simulink model "kfs_pr_1"  (R2019a)
settings: Solver=FixedStepAuto  StartTime=0.0  StopTime=10000  FixedStep=1  RelTol=1e-3
values from neighbouring files (symbols this model uses):
  mb = 10800    [params.m]
  min_paus = 100    [params.m]
  nurk = deg2rad(0)    [params.m]
  vy_0 = 0    [params.m]
  x_0 = 0    [params.m]
  y_0 = 0    [params.m]
libraries: dspswit3 x1, simulink x1
settings Model: Creator=Kasutaja  LastModifiedBy=Kasutaja
settings DataIOCC: ReturnWorkspaceOutputs=off
settings DebuggingCC: ArithmeticOperatorsInVariantConditions=warning

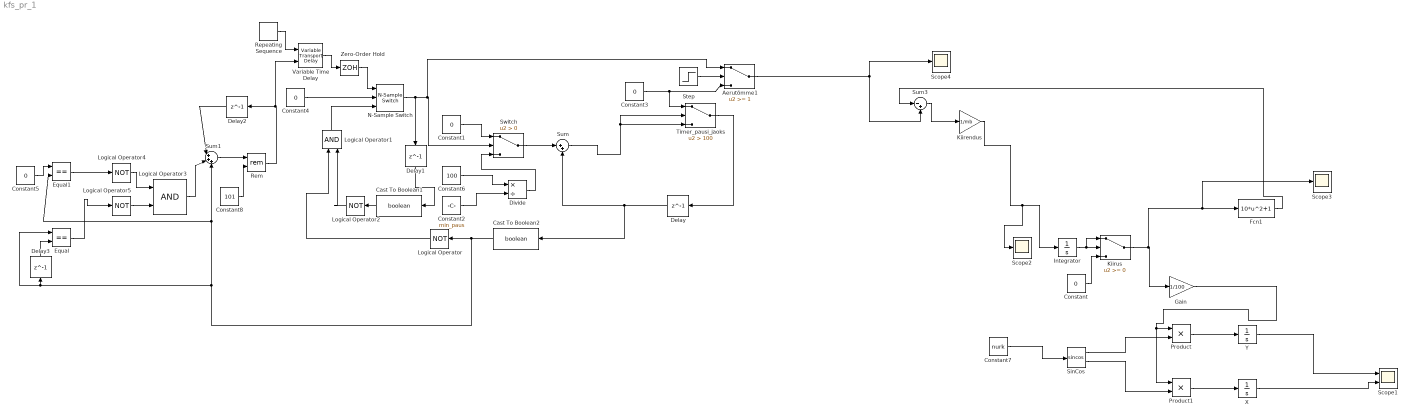
== system kfs_pr_1 ==
  Aerutõmme1 : Switch  Threshold=1
  Cast To Boolean1 : DataTypeConversion  OutDataTypeStr=boolean
  Cast To Boolean2 : DataTypeConversion  OutDataTypeStr=boolean
  Constant{,1,3..5} (5 alike) : Constant  Value=0
  Constant2 : Constant  Value=min_paus  SampleTime=1
  Constant6 : Constant  Value=100  SampleTime=1
  Constant7 : Constant  Value=nurk
  Constant8 : Constant  Value=101
  Delay{,1..3} (4 alike) : Delay  DelayLength=1  InitialCondition=0
  Divide : Product  Inputs=*/
  Equal : RelationalOperator  Operator===  OutDataTypeStr=boolean  RndMeth=Simplest
  Equal1 : RelationalOperator  Operator===  OutDataTypeStr=boolean  RndMeth=Simplest
  Fcn1 : Fcn  Expr=10*u^2+1
  Gain : Gain  Gain=1/100
  Integrator : Integrator  InitialCondition=vy_0
  Kiirendus : Gain  Gain=1/mb
  Kiirus : Switch
  Logical Operator{,2,4..5} (4 alike) : Logic  Operator=NOT  IconShape=distinctive  AllPortsSameDT=off  OutDataTypeStr=boolean
  Logical Operator1 : Logic  IconShape=distinctive  AllPortsSameDT=off  OutDataTypeStr=boolean
  Logical Operator3 : Logic  IconShape=distinctive  AllPortsSameDT=off  OutDataTypeStr=boolean
  N-Sample Switch : dspswit3/N-Sample Switch  N=101  reset=on  TriggerType=Non-zero sample  Ts=1
      settings: SourceProductName=DSP System Toolbox  SourceProductBaseCode=DS
  Product : Product
  Product1 : Product
  Rem : Math  Operator=rem  SaturateOnIntegerOverflow=on
  Repeating Sequence : simulink/Sources/Repeating Sequence  rep_seq_t=|  rep_seq_y=|
      rep_seq_t=|
      | [0
      | 1
      | 2
      | 3
      | 4
      | 5
      | 6
      | 7
      | 8
      | 9
      | 10
      | 11
      | 12
      | 13
      | 14
      | 15
      | 16
      | 17
      | 18
      | 19
      | 20
      | 21
      | 22
      | 23
      | 24
      | 25
      | 26
      | 27
      | 28
      | 29
      | 30
      | 31
      | 32
      | 33
      | 34
      | 35
      | 36
      | 37
      | 38
      | 39
      | 40
      | 41
      | 42
      | 43
      | 44
      | 45
      | 46
      | 47
      | 48
      | 49
      | 50
      | 51
      | 52
      | 53
      | 54
      | 55
      | 56
      | 57
      | 58
      | 59
      | 60
      | 61
      | 62
      | 63
      | 64
      | 65
      | 66
      | 67
      | 68
      | 69
      | 70
      | 71
      | 72
      | 73
      | 74
      | 75
      | 76
      | 77
      | 78
      | 79
      | 80
      | 81
      | 82
      | 83
      | 84
      | 85
      | 86
      | 87
      | 88
      | 89
      | 90
      | 91
      | 92
      | 93
      | 94
      | 95
      | 96
      | 97
      | 98
      | 99
      | 100
      | 101  ]
      rep_seq_y=|
      | [1
      | 14
      | 28
      | 42
      | 56
      | 70
      | 84
      | 98
      | 112
      | 126
      | 167
      | 208
      | 249
      | 290
      | 331
      | 372
      | 413
      | 454
      | 495
      | 536
      | 551
      | 566
      | 581
      | 596
      | 611
      | 626
      | 641
      | 656
      | 671
      | 686
      | 697
      | 708
      | 719
      | 730
      | 741
      | 752
      | 763
      | 774
      | 785
      | 796
      | 801
      | 806
      | 811
      | 816
      | 821
      | 826
      | 831
      | 836
      | 841
      | 846
      | 841
      | 836
      | 831
      | 826
      | 821
      | 816
      | 811
      | 806
      | 801
      | 796
      | 785
      | 774
      | 763
      | 752
      | 741
      | 730
      | 719
      | 708
      | 697
      | 686
      | 646
      | 606
      | 566
      | 526
      | 486
      | 446
      | 406
      | 366
      | 326
      | 286
      | 279
      | 272
      | 265
      | 258
      | 251
      | 244
      | 237
      | 230
      | 223
      | 216
      | 198
      | 180
      | 162
      | 144
      | 126
      | 108
      | 90
      | 72
      | 54
      | 36
      | 18
      | -1  ]
  Scope1 : Scope  NumInputPorts=2
  Scope2 : Scope
  Scope3 : Scope
  Scope4 : Scope
  SinCos : Trigonometry  Operator=sincos
  Step : Step  Time=2000  Before=1  After=0  SampleTime=1
  Sum : Sum  Inputs=|++
  Sum1 : Sum  Inputs=|+++
  Sum3 : Sum  Inputs=|-+
  Switch : Switch  Criteria=u2 > Threshold
  Timer_pausi_jaoks : Switch  Criteria=u2 > Threshold  Threshold=100
  Variable Time Delay : VariableTransportDelay  MaximumDelay=200  MaximumPoints=256  ZeroDelay=on
  X : Integrator  InitialCondition=x_0
  Y : Integrator  InitialCondition=y_0
  Zero-Order Hold : ZeroOrderHold
  wires:
  Aerutõmme1/1 -> Sum3/2, Scope4/1
  X/1 -> Scope1/2
  Fcn1/1 -> Sum3/1
  Y/1 -> Scope1/1
  Product1/1 -> X/1
  Constant7/1 -> SinCos/1
  Kiirendus/1 -> Integrator/1, Scope2/1
  SinCos/1 -> Product/2
  SinCos/2 -> Product1/2
  Product/1 -> Y/1
  Gain/1 -> Product1/1, Product/1
  Sum3/1 -> Kiirendus/1
  Cast To Boolean2/1 -> Sum1/3, Equal1/2, Delay3/1, Equal/1, Logical Operator/1
  Constant6/1 -> Divide/1
  Constant5/1 -> Equal1/1
  Logical Operator1/1 -> N-Sample Switch/3
  Constant1/1 -> Switch/1
  Zero-Order Hold/1 -> N-Sample Switch/1
  Repeating Sequence/1 -> Variable Time Delay/1
  Logical Operator5/1 -> Logical Operator3/2
  Constant3/1 -> Aerutõmme1/3, Timer_pausi_jaoks/1
  Delay1/1 -> Cast To Boolean1/1
  Constant2/1 -> Divide/2
  Logical Operator3/1 -> Sum1/2
  Delay/1 -> Cast To Boolean2/1, Sum/2
  Equal/1 -> Logical Operator5/1
  Step/1 -> Aerutõmme1/2
  Timer_pausi_jaoks/1 -> Delay/1
  Delay3/1 -> Equal/2
  Sum/1 -> Timer_pausi_jaoks/3, Timer_pausi_jaoks/2
  Sum1/1 -> Rem/1
  Divide/1 -> Switch/3
  Delay2/1 -> Sum1/1
  Equal1/1 -> Logical Operator4/1
  Logical Operator/1 -> Logical Operator1/1
  Constant4/1 -> N-Sample Switch/2
  Switch/1 -> Sum/1
  Logical Operator4/1 -> Logical Operator3/1
  Logical Operator2/1 -> Logical Operator1/2
  Cast To Boolean1/1 -> Logical Operator2/1
  Kiirus/1 -> Scope3/1, Fcn1/1, Gain/1
  Integrator/1 -> Kiirus/1, Kiirus/2
  Constant/1 -> Kiirus/3
  Rem/1 -> Variable Time Delay/2, Delay2/1
  Constant8/1 -> Rem/2
  Variable Time Delay/1 -> Zero-Order Hold/1
  N-Sample Switch/1 -> Aerutõmme1/1, Switch/2, Delay1/1
